simulink model "DLCReferenceApplication"  (R2018a)
settings: Solver=ode23tb  StartTime=0.0  StopTime=20  FixedStep=.001  RelTol=5e-3  EnableMultiTasking=on
StartFcn:
  | %tic
StopFcn:
  | %toc
model workspace (MAT data in the model file):
  A_mu = 10
  B_reff = 8.386
  Cz = 7766.25
  DCT_Param : struct (value not decoded)
  D_reff = 0.25826
  Downshift_Speeds = [9.5625 12.9375 16.3125 19.6875 23.0625 26.4375 29.8125 33.1875 36.5625 39.9375 43.3125 46.6875 ... (28 elements, 4x7)]
  Pedal_Positions = [0.1 0.4 0.5 0.9]
  SUS : struct (value not decoded)
  Upshift_Speeds = [12.9375 16.3125 19.6875 33 26.4375 29.8125 33.1875 52.5 39.9375 43.3125 46.6875 77.25 ... (28 elements, 4x7)]
  VEH : struct (value not decoded)
  V_o = 16.7
  V_xlow = 1
  WH : struct (value not decoded)
  a = 1.4
  alpha_max = 1.5
  alpha_min = -1.5
  b = 1.8
  c_zo = 209651
  epsilon = 0.1
  h = 0.134
  path : struct (value not decoded)
  pio = 220000
  q_Fcx = 0
  q_Fz2 = 15.4
  q_Fzy = 0
  q_reo = 0.9974
  q_sx1 = -0.007764
  q_sx10 = 0.2824
  q_sx11 = 5.349
  q_sx12 = 0
  q_sx13 = 0
  q_sx14 = 0
  q_sx2 = 1.1915
  q_sx3 = 0.013948
  q_sx4 = 4.912
  q_sx5 = 1.02
  q_sx6 = 22.83
  q_sx7 = 0.7104
  q_sx8 = -0.023393
  q_sx9 = 0.6581
  q_sy1 = 0.00702
  q_sy2 = 0
  q_sy3 = 0.001515
  q_sy4 = 8.514e-05
  q_sy5 = 0
  q_sy6 = 0
  q_sy7 = 0.9008
  q_sy8 = -0.4089
  q_v1 = 0.0007742
  q_v2 = 0.04667
  r_Bx1 = 12.531
  r_Bx2 = 9.532
  r_Bx3 = 0
  r_By1 = 10.615
  r_By2 = 7.705
  r_By3 = 3.433e-06
  r_By4 = 0
  r_Cx1 = 1.019
  r_Cy1 = 1.0585
  r_Ex1 = -0.4487
  r_Ex2 = -0.4726
  r_Ey1 = 0.3132
  r_Ey2 = 7.63e-06
  r_Hx1 = 0.0002374
  r_Hy1 = 0.011646
  r_Hy2 = 7.63e-06
  r_Vy1 = 0.05654
  r_Vy2 = 7.63e-06
  r_Vy3 = 0
  r_Vy4 = 99.9
  r_Vy5 = 2
  r_Vy6 = 15.814
  r_o = 0.3135
  vehWidth = 2
  w = 1
symbols that are objects in the model workspace (value not decoded): VEH
libraries: neural x286, simulink x5, sim3dlib x2, autolibutils x1, vehdynlibscenariocommon x1, vehdynlibdriver x1, vehdynlibviscommon x1
(part 3 of 13)

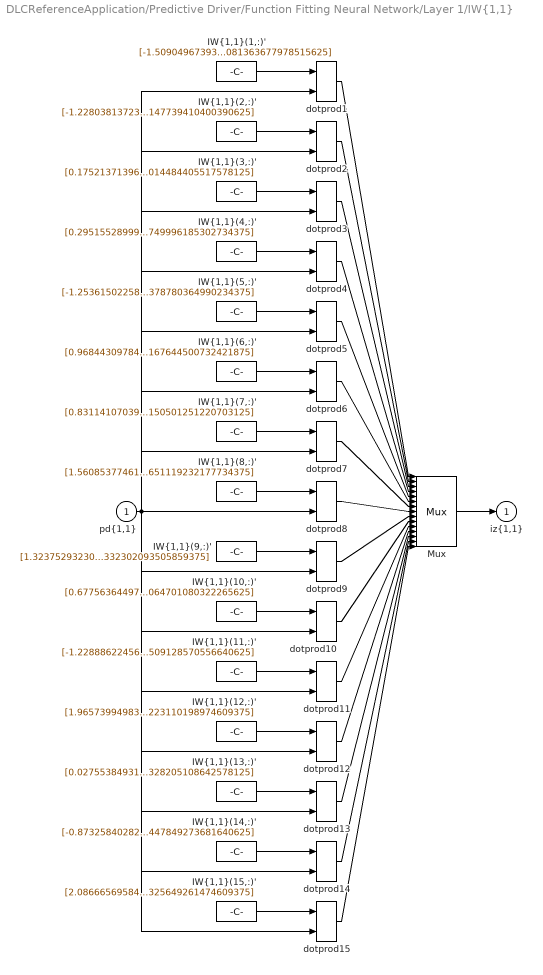
== system DLCReferenceApplication/Predictive Driver/Function Fitting Neural Network/Layer 1/IW{1,1} ==
  "pd{1,1}" : Inport  PortDimensions=7
      mask Display: e = 0.06;c1 = [120 230 180]/255;c2 = ([120 230 180]+0)/(256+128);c3 = ([120 230 180]+128)/(256+128);patch([0 1 1 0],[0 0 1 1],c1);patch([0 1 1 1-e 1-e 0+e],[0 0 1 1-e 0+e 0+e],c2);patch([0 0 1 1-e 0+e 0+e],[0 1 1 1-e 1-e 0+e],c3);plot([0 1 1 0 0],[0 0 1 1 0]);
  "IW{1,1}(1,:)'" : Constant  Value=[-1.509049673932340684956443510600365698337554931640625;1.51927734183694784775298103340901434421539306640625;1.479181269120346531309451165725477039813995361328125;0.76292036319028133650732570458785630762577056884765625;-1.4000753923386464183664656957262195646762847900390625;1.516189767355066830845089498325251042842864990234375;-0.6979172108090470061370069743134081363677978515625]
      mask Display: e = 0.06;c1 = [120 150 230]/255;c2 = ([120 150 230]+0)/383;c3 = ([120 150 230]+128)/383;patch([0 1 1 0],[0 0 1 1],c1);patch([0 1 1 1-e 1-e 0+e],[0 0 1 1-e 0+e 0+e],c2);patch([0 0 1 1-e 0+e 0+e],[0 1 1 1-e 1-e 0+e],c3);plot([0 1 1 0 0],[0 0 1 1 0]);disp('Weights');
  "IW{1,1}(10,:)'" : Constant  Value=[0.67756364497310739292146308798692189157009124755859375;0.04182033064572175662387820693766116164624691009521484375;-0.4504897562480543182772407817537896335124969482421875;-2.551876443899323110287014060304500162601470947265625;0.18672185850221978409280154664884321391582489013671875;1.7325835923135628480196146483649499714374542236328125;0.289998821125625971806272218600497581064701080322265625]
      mask Display: e = 0.06;c1 = [120 150 230]/255;c2 = ([120 150 230]+0)/383;c3 = ([120 150 230]+128)/383;patch([0 1 1 0],[0 0 1 1],c1);patch([0 1 1 1-e 1-e 0+e],[0 0 1 1-e 0+e 0+e],c2);patch([0 0 1 1-e 0+e 0+e],[0 1 1 1-e 1-e 0+e],c3);plot([0 1 1 0 0],[0 0 1 1 0]);disp('Weights');
  "IW{1,1}(11,:)'" : Constant  Value=[-1.2288862245678371376556015093228779733180999755859375;-0.70363000734339908870396129714208655059337615966796875;-1.5288499399296260339298214603331871330738067626953125;-1.1174320519343565738523693653405643999576568603515625;1.6750447749892007909267022114363498985767364501953125;-2.4972953199852252481605319189839065074920654296875;0.70182493954114166800906104981550015509128570556640625]
      mask Display: e = 0.06;c1 = [120 150 230]/255;c2 = ([120 150 230]+0)/383;c3 = ([120 150 230]+128)/383;patch([0 1 1 0],[0 0 1 1],c1);patch([0 1 1 1-e 1-e 0+e],[0 0 1 1-e 0+e 0+e],c2);patch([0 0 1 1-e 0+e 0+e],[0 1 1 1-e 1-e 0+e],c3);plot([0 1 1 0 0],[0 0 1 1 0]);disp('Weights');
  "IW{1,1}(12,:)'" : Constant  Value=[1.9657399498320062836143051754334010183811187744140625;0.055469671143939518198617832922536763362586498260498046875;0.428893001178795640893071094978949986398220062255859375;0.83038703202997699026610689543304033577442169189453125;0.6528646345537374440226585647906176745891571044921875;-1.7892558675957606073581018790719099342823028564453125;-1.87816849195586765830512376851402223110198974609375]
      mask Display: e = 0.06;c1 = [120 150 230]/255;c2 = ([120 150 230]+0)/383;c3 = ([120 150 230]+128)/383;patch([0 1 1 0],[0 0 1 1],c1);patch([0 1 1 1-e 1-e 0+e],[0 0 1 1-e 0+e 0+e],c2);patch([0 0 1 1-e 0+e 0+e],[0 1 1 1-e 1-e 0+e],c3);plot([0 1 1 0 0],[0 0 1 1 0]);disp('Weights');
  "IW{1,1}(13,:)'" : Constant  Value=[0.027553849311181564940564925336730084381997585296630859375;0.165556284993658930915216842549853026866912841796875;1.0787466889472050457499108233605511486530303955078125;-1.89957440383020159657689873711206018924713134765625;0.54115146920791890039481586427427828311920166015625;-1.653817387983281150809489190578460693359375;1.1876738967274527158934915860299952328205108642578125]
      mask Display: e = 0.06;c1 = [120 150 230]/255;c2 = ([120 150 230]+0)/383;c3 = ([120 150 230]+128)/383;patch([0 1 1 0],[0 0 1 1],c1);patch([0 1 1 1-e 1-e 0+e],[0 0 1 1-e 0+e 0+e],c2);patch([0 0 1 1-e 0+e 0+e],[0 1 1 1-e 1-e 0+e],c3);plot([0 1 1 0 0],[0 0 1 1 0]);disp('Weights');
  "IW{1,1}(14,:)'" : Constant  Value=[-0.873258402827774116161663187085650861263275146484375;2.211312160674173465935155036277137696743011474609375;-2.483318885241498463756215642206370830535888671875;2.537018816534186260724936801125295460224151611328125;2.2595527875997465372392980498261749744415283203125;-4.12440023174638614733567010262049734592437744140625;2.3447201728720248325998909422196447849273681640625]
      mask Display: e = 0.06;c1 = [120 150 230]/255;c2 = ([120 150 230]+0)/383;c3 = ([120 150 230]+128)/383;patch([0 1 1 0],[0 0 1 1],c1);patch([0 1 1 1-e 1-e 0+e],[0 0 1 1-e 0+e 0+e],c2);patch([0 0 1 1-e 0+e 0+e],[0 1 1 1-e 1-e 0+e],c3);plot([0 1 1 0 0],[0 0 1 1 0]);disp('Weights');
  "IW{1,1}(15,:)'" : Constant  Value=[2.08666569584865957409647307940758764743804931640625;-0.80442585468800620329687944831675849854946136474609375;-0.379133263113434482161068217465071938931941986083984375;-0.2375698497917715368288327226764522492885589599609375;0.10421540704451726089274643527460284531116485595703125;-0.77514844988269893111265673724119551479816436767578125;0.3039233762085336021385728599852882325649261474609375]
      mask Display: e = 0.06;c1 = [120 150 230]/255;c2 = ([120 150 230]+0)/383;c3 = ([120 150 230]+128)/383;patch([0 1 1 0],[0 0 1 1],c1);patch([0 1 1 1-e 1-e 0+e],[0 0 1 1-e 0+e 0+e],c2);patch([0 0 1 1-e 0+e 0+e],[0 1 1 1-e 1-e 0+e],c3);plot([0 1 1 0 0],[0 0 1 1 0]);disp('Weights');
  "IW{1,1}(2,:)'" : Constant  Value=[-1.22803813723280175196350683108903467655181884765625;-2.25896918882737285372286351048387587070465087890625;-0.4219079312453886121403456854750402271747589111328125;-1.695805476122420163420656535890884697437286376953125;1.6764860652005861840763145664823241531848907470703125;-0.288104929415635313549870488714077509939670562744140625;1.1836646212486352514048348893993534147739410400390625]
      mask Display: e = 0.06;c1 = [120 150 230]/255;c2 = ([120 150 230]+0)/383;c3 = ([120 150 230]+128)/383;patch([0 1 1 0],[0 0 1 1],c1);patch([0 1 1 1-e 1-e 0+e],[0 0 1 1-e 0+e 0+e],c2);patch([0 0 1 1-e 0+e 0+e],[0 1 1 1-e 1-e 0+e],c3);plot([0 1 1 0 0],[0 0 1 1 0]);disp('Weights');
  "IW{1,1}(3,:)'" : Constant  Value=[0.17521371396843898882167422925704158842563629150390625;-1.5068324243738988599261574563570320606231689453125;-0.339896798386482734688485152219072915613651275634765625;1.2475380308633063908274607456405647099018096923828125;3.277106824369047100020679863519035279750823974609375;0.1745122092133344626763147289238986559212207794189453125;-2.210738215368686088169170034234412014484405517578125]
      mask Display: e = 0.06;c1 = [120 150 230]/255;c2 = ([120 150 230]+0)/383;c3 = ([120 150 230]+128)/383;patch([0 1 1 0],[0 0 1 1],c1);patch([0 1 1 1-e 1-e 0+e],[0 0 1 1-e 0+e 0+e],c2);patch([0 0 1 1-e 0+e 0+e],[0 1 1 1-e 1-e 0+e],c3);plot([0 1 1 0 0],[0 0 1 1 0]);disp('Weights');
  "IW{1,1}(4,:)'" : Constant  Value=[0.295155289995136682623666501967818476259708404541015625;0.54169014463003517523276286738109774887561798095703125;-0.81923187750457915345947412788518704473972320556640625;-1.413502828991773707656420810963027179241180419921875;0.7249327311390978412219965321128256618976593017578125;0.25822608938690316815467440392239950597286224365234375;3.05246104088644099050497970893047749996185302734375]
      mask Display: e = 0.06;c1 = [120 150 230]/255;c2 = ([120 150 230]+0)/383;c3 = ([120 150 230]+128)/383;patch([0 1 1 0],[0 0 1 1],c1);patch([0 1 1 1-e 1-e 0+e],[0 0 1 1-e 0+e 0+e],c2);patch([0 0 1 1-e 0+e 0+e],[0 1 1 1-e 1-e 0+e],c3);plot([0 1 1 0 0],[0 0 1 1 0]);disp('Weights');
  "IW{1,1}(5,:)'" : Constant  Value=[-1.253615022589892991078386330627836287021636962890625;-1.308178888292455877007114395382814109325408935546875;-0.55746399823290404551556775913923047482967376708984375;2.888853599694045204415715488721616566181182861328125;0.67366408192522564402082707601948641240596771240234375;1.7511351672237738252846384057193063199520111083984375;-0.550561400887894958344759288593195378780364990234375]
      mask Display: e = 0.06;c1 = [120 150 230]/255;c2 = ([120 150 230]+0)/383;c3 = ([120 150 230]+128)/383;patch([0 1 1 0],[0 0 1 1],c1);patch([0 1 1 1-e 1-e 0+e],[0 0 1 1-e 0+e 0+e],c2);patch([0 0 1 1-e 0+e 0+e],[0 1 1 1-e 1-e 0+e],c3);plot([0 1 1 0 0],[0 0 1 1 0]);disp('Weights');
  "IW{1,1}(6,:)'" : Constant  Value=[0.968443097846008793538885583984665572643280029296875;-1.02085143200877492830613846308551728725433349609375;-2.7100181628849835391292799613438546657562255859375;-1.469426684764355339751773499301634728908538818359375;-0.72093283243393291304101921923574991524219512939453125;0.0298446565267905077056820317693563993088901042938232421875;0.2776436857395701007789057257468812167644500732421875]
      mask Display: e = 0.06;c1 = [120 150 230]/255;c2 = ([120 150 230]+0)/383;c3 = ([120 150 230]+128)/383;patch([0 1 1 0],[0 0 1 1],c1);patch([0 1 1 1-e 1-e 0+e],[0 0 1 1-e 0+e 0+e],c2);patch([0 0 1 1-e 0+e 0+e],[0 1 1 1-e 1-e 0+e],c3);plot([0 1 1 0 0],[0 0 1 1 0]);disp('Weights');
  "IW{1,1}(7,:)'" : Constant  Value=[0.83114107039691231815226046819589100778102874755859375;-1.653778663789594371991142907063476741313934326171875;1.7070538673297175336074360529892146587371826171875;-0.467894735272818274030015572861884720623493194580078125;-1.4874423762862181153110441300668753683567047119140625;0.1529353896317520999925676505881710909307003021240234375;-0.51792644395898801423783197606098838150501251220703125]
      mask Display: e = 0.06;c1 = [120 150 230]/255;c2 = ([120 150 230]+0)/383;c3 = ([120 150 230]+128)/383;patch([0 1 1 0],[0 0 1 1],c1);patch([0 1 1 1-e 1-e 0+e],[0 0 1 1-e 0+e 0+e],c2);patch([0 0 1 1-e 0+e 0+e],[0 1 1 1-e 1-e 0+e],c3);plot([0 1 1 0 0],[0 0 1 1 0]);disp('Weights');
  "IW{1,1}(8,:)'" : Constant  Value=[1.5608537746191044615073906243196688592433929443359375;0.8208342730039908108352619819925166666507720947265625;1.70216863375625049314976422465406358242034912109375;-0.95886390034983914887334321974776685237884521484375;3.42297237946134469410708334180526435375213623046875;0.6162829570883274765691339780460111796855926513671875;3.2692680483829601456591262831352651119232177734375]
      mask Display: e = 0.06;c1 = [120 150 230]/255;c2 = ([120 150 230]+0)/383;c3 = ([120 150 230]+128)/383;patch([0 1 1 0],[0 0 1 1],c1);patch([0 1 1 1-e 1-e 0+e],[0 0 1 1-e 0+e 0+e],c2);patch([0 0 1 1-e 0+e 0+e],[0 1 1 1-e 1-e 0+e],c3);plot([0 1 1 0 0],[0 0 1 1 0]);disp('Weights');
  "IW{1,1}(9,:)'" : Constant  Value=[1.3237529323020209570671568144462071359157562255859375;-0.44844324720964079400431501198909245431423187255859375;-3.795885956504914116038662541541270911693572998046875;-1.1322778939762268013424773016595281660556793212890625;-0.50600361676503669006166319377371110022068023681640625;-1.3597783903850106934640962208504788577556610107421875;-1.599955115091173496466581127606332302093505859375]
      mask Display: e = 0.06;c1 = [120 150 230]/255;c2 = ([120 150 230]+0)/383;c3 = ([120 150 230]+128)/383;patch([0 1 1 0],[0 0 1 1],c1);patch([0 1 1 1-e 1-e 0+e],[0 0 1 1-e 0+e 0+e],c2);patch([0 0 1 1-e 0+e 0+e],[0 1 1 1-e 1-e 0+e],c3);plot([0 1 1 0 0],[0 0 1 1 0]);disp('Weights');
  Mux : Mux  Inputs=15
      mask Display: e = 0.06;c1 = [120 150 230]/255;c2 = ([120 150 230]+0)/383;c3 = ([120 150 230]+128)/383;patch([0 1 1 0],[0 0 1 1],c1);patch([0 1 1 1-e 1-e 0+e],[0 0 1 1-e 0+e 0+e],c2);patch([0 0 1 1-e 0+e 0+e],[0 1 1 1-e 1-e 0+e],c3);plot([0 1 1 0 0],[0 0 1 1 0]);disp('Mux');
  dotprod{1..15} (15 alike) : neural/Weight Functions/dotprod
  "iz{1,1}" : Outport
      mask Display: e = 0.06;c1 = [120 230 180]/255;c2 = ([120 230 180]+0)/(256+128);c3 = ([120 230 180]+128)/(256+128);patch([0 1 1 0],[0 0 1 1],c1);patch([0 1 1 1-e 1-e 0+e],[0 0 1 1-e 0+e 0+e],c2);patch([0 0 1 1-e 0+e 0+e],[0 1 1 1-e 1-e 0+e],c3);plot([0 1 1 0 0],[0 0 1 1 0]);
  wires:
  "IW{1,1}(1,:)'"/1 -> dotprod1/1
  "pd{1,1}"/1 -> dotprod1/2, dotprod2/2, dotprod3/2, dotprod4/2, dotprod5/2, dotprod6/2, dotprod7/2, dotprod8/2, dotprod9/2, dotprod10/2, dotprod11/2, dotprod12/2, dotprod13/2, dotprod14/2, dotprod15/2
  dotprod1/1 -> Mux/1
  "IW{1,1}(2,:)'"/1 -> dotprod2/1
  dotprod2/1 -> Mux/2
  "IW{1,1}(3,:)'"/1 -> dotprod3/1
  dotprod3/1 -> Mux/3
  "IW{1,1}(4,:)'"/1 -> dotprod4/1
  dotprod4/1 -> Mux/4
  "IW{1,1}(5,:)'"/1 -> dotprod5/1
  dotprod5/1 -> Mux/5
  "IW{1,1}(6,:)'"/1 -> dotprod6/1
  dotprod6/1 -> Mux/6
  "IW{1,1}(7,:)'"/1 -> dotprod7/1
  dotprod7/1 -> Mux/7
  "IW{1,1}(8,:)'"/1 -> dotprod8/1
  dotprod8/1 -> Mux/8
  "IW{1,1}(9,:)'"/1 -> dotprod9/1
  dotprod9/1 -> Mux/9
  "IW{1,1}(10,:)'"/1 -> dotprod10/1
  dotprod10/1 -> Mux/10
  "IW{1,1}(11,:)'"/1 -> dotprod11/1
  dotprod11/1 -> Mux/11
  "IW{1,1}(12,:)'"/1 -> dotprod12/1
  dotprod12/1 -> Mux/12
  "IW{1,1}(13,:)'"/1 -> dotprod13/1
  dotprod13/1 -> Mux/13
  "IW{1,1}(14,:)'"/1 -> dotprod14/1
  dotprod14/1 -> Mux/14
  "IW{1,1}(15,:)'"/1 -> dotprod15/1
  dotprod15/1 -> Mux/15
  Mux/1 -> "iz{1,1}"/1

== system DLCReferenceApplication/Predictive Driver/Function Fitting Neural Network/Layer 2/Delays 1 ==
  "p{2}" : Inport  PortDimensions=15
      mask Display: e = 0.06;c1 = [120 230 180]/255;c2 = ([120 230 180]+0)/(256+128);c3 = ([120 230 180]+128)/(256+128);patch([0 1 1 0],[0 0 1 1],c1);patch([0 1 1 1-e 1-e 0+e],[0 0 1 1-e 0+e 0+e],c2);patch([0 0 1 1-e 0+e 0+e],[0 1 1 1-e 1-e 0+e],c3);plot([0 1 1 0 0],[0 0 1 1 0]);
  mux : Mux  Inputs=1
      mask Display: e = 0.06;c1 = [120 150 230]/255;c2 = ([120 150 230]+0)/383;c3 = ([120 150 230]+128)/383;patch([0 1 1 0],[0 0 1 1],c1);patch([0 1 1 1-e 1-e 0+e],[0 0 1 1-e 0+e 0+e],c2);patch([0 0 1 1-e 0+e 0+e],[0 1 1 1-e 1-e 0+e],c3);plot([0 1 1 0 0],[0 0 1 1 0]);disp('Mux')
  "pd{2,1}" : Outport
      mask Display: e = 0.06;c1 = [120 230 180]/255;c2 = ([120 230 180]+0)/(256+128);c3 = ([120 230 180]+128)/(256+128);patch([0 1 1 0],[0 0 1 1],c1);patch([0 1 1 1-e 1-e 0+e],[0 0 1 1-e 0+e 0+e],c2);patch([0 0 1 1-e 0+e 0+e],[0 1 1 1-e 1-e 0+e],c3);plot([0 1 1 0 0],[0 0 1 1 0]);
  wires:
  "p{2}"/1 -> mux/1
  mux/1 -> "pd{2,1}"/1

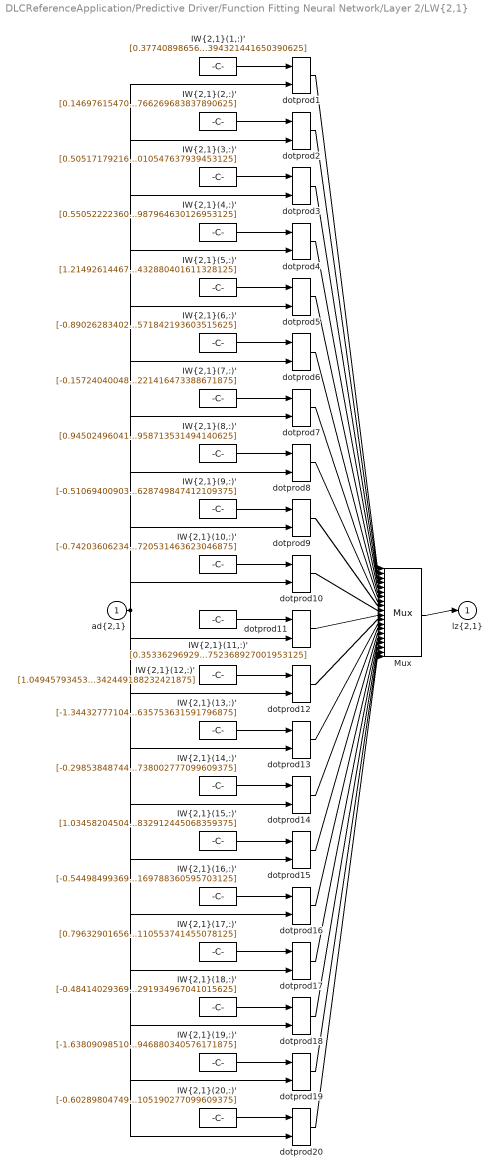
== system DLCReferenceApplication/Predictive Driver/Function Fitting Neural Network/Layer 2/LW{2,1} ==
  "ad{2,1}" : Inport  PortDimensions=15
      mask Display: e = 0.06;c1 = [120 230 180]/255;c2 = ([120 230 180]+0)/(256+128);c3 = ([120 230 180]+128)/(256+128);patch([0 1 1 0],[0 0 1 1],c1);patch([0 1 1 1-e 1-e 0+e],[0 0 1 1-e 0+e 0+e],c2);patch([0 0 1 1-e 0+e 0+e],[0 1 1 1-e 1-e 0+e],c3);plot([0 1 1 0 0],[0 0 1 1 0]);
  "IW{2,1}(1,:)'" : Constant  Value=[0.377408986567094262287724859561421908438205718994140625;0.916935828034818545262396582984365522861480712890625;0.393088948975864271861979659661301411688327789306640625;-0.6492111185444693344237521159811876714229583740234375;-0.203739226760496883184003991118515841662883758544921875;-0.1100086759278134651562908175037591718137264251708984375;0.351124696378162237664355416200123727321624755859375;0.540735910832136124071212179842405021190643310546875;-0.52499617358879613338018543799989856779575347900390625;-0.8542847095270953428070015434059314429759979248046875;0.7305202305645150939739096429548226296901702880859375;0.26047154767623614812777077531791292130947113037109375;-0.5187381603465672785802098587737418711185455322265625;0.11664270786766640919385196184521191753447055816650390625;-0.374314853750083609273957563345902599394321441650390625]
      mask Display: e = 0.06;c1 = [120 150 230]/255;c2 = ([120 150 230]+0)/383;c3 = ([120 150 230]+128)/383;patch([0 1 1 0],[0 0 1 1],c1);patch([0 1 1 1-e 1-e 0+e],[0 0 1 1-e 0+e 0+e],c2);patch([0 0 1 1-e 0+e 0+e],[0 1 1 1-e 1-e 0+e],c3);plot([0 1 1 0 0],[0 0 1 1 0]);disp('weights');
  "IW{2,1}(10,:)'" : Constant  Value=[-0.74203606234167496236153738209395669400691986083984375;-0.812696026932474335779943430679850280284881591796875;-0.6131789681735482222535438268096186220645904541015625;0.1180891377801421004978266182661172933876514434814453125;0.397427019878926424123477545435889624059200286865234375;2.659200302624636691462001181207597255706787109375;0.8379336594029853646503624986507929861545562744140625;-0.51262919422646213707395190795068629086017608642578125;-0.2688533984134124921183683909475803375244140625;0.7557158363858416105784954197588376700878143310546875;-0.492959648338735345607375393228721804916858673095703125;0.0773063422443649173043667133242706768214702606201171875;-0.406745691526066044385601117028272710740566253662109375;-0.7792669239456808671917542596929706633090972900390625;0.6259901693968170643955772902700118720531463623046875]
      mask Display: e = 0.06;c1 = [120 150 230]/255;c2 = ([120 150 230]+0)/383;c3 = ([120 150 230]+128)/383;patch([0 1 1 0],[0 0 1 1],c1);patch([0 1 1 1-e 1-e 0+e],[0 0 1 1-e 0+e 0+e],c2);patch([0 0 1 1-e 0+e 0+e],[0 1 1 1-e 1-e 0+e],c3);plot([0 1 1 0 0],[0 0 1 1 0]);disp('weights');
  "IW{2,1}(11,:)'" : Constant  Value=[0.3533629692989530557412081179791130125522613525390625;-0.81541740940325035946756315752281807363033294677734375;-2.0683095123156203243297568405978381633758544921875;0.35160466105935561653694776396150700747966766357421875;0.47449346143949344689616509640472941100597381591796875;1.85236410264457074248412027372978627681732177734375;-0.81173488668558591019319692350109107792377471923828125;-0.8655341239549638743255854933522641658782958984375;0.54966802080016818887742147126118652522563934326171875;0.0288250527353895273641182228629986639134585857391357421875;-0.51036540540294594858750087951193563640117645263671875;-0.040133000774815463795874848074163310229778289794921875;-0.89000331812890742799737608947907574474811553955078125;0.678463611178770964471596016664989292621612548828125;0.04549854251039338326467742490422097034752368927001953125]
      mask Display: e = 0.06;c1 = [120 150 230]/255;c2 = ([120 150 230]+0)/383;c3 = ([120 150 230]+128)/383;patch([0 1 1 0],[0 0 1 1],c1);patch([0 1 1 1-e 1-e 0+e],[0 0 1 1-e 0+e 0+e],c2);patch([0 0 1 1-e 0+e 0+e],[0 1 1 1-e 1-e 0+e],c3);plot([0 1 1 0 0],[0 0 1 1 0]);disp('weights');
  "IW{2,1}(12,:)'" : Constant  Value=[1.0494579345300130146512174178496934473514556884765625;1.3044889644552188912030032952316105365753173828125;-0.27106298353604463269306279471493326127529144287109375;-0.1915871026849610692099901143592433072626590728759765625;-0.34760653690221354761291649992926977574825286865234375;0.52037978849581134621615774449310265481472015380859375;-0.2321169942446153766635319470879039727151393890380859375;0.332861282582828821308140732071478851139545440673828125;-1.3938611465836869829360011863172985613346099853515625;0.8212779725642869177448801565333269536495208740234375;0.1046906705946868132439675491696107201278209686279296875;-0.30151606216337956123396679686265997588634490966796875;0.4956805530473360477117239497601985931396484375;-0.71076779296117820194922387599945068359375;-0.48071803830861703499266468497808091342449188232421875]
      mask Display: e = 0.06;c1 = [120 150 230]/255;c2 = ([120 150 230]+0)/383;c3 = ([120 150 230]+128)/383;patch([0 1 1 0],[0 0 1 1],c1);patch([0 1 1 1-e 1-e 0+e],[0 0 1 1-e 0+e 0+e],c2);patch([0 0 1 1-e 0+e 0+e],[0 1 1 1-e 1-e 0+e],c3);plot([0 1 1 0 0],[0 0 1 1 0]);disp('weights');
  "IW{2,1}(13,:)'" : Constant  Value=[-1.344327771042938213241768607986159622669219970703125;-0.349408651716258733532782798647531308233737945556640625;-0.390264497355393424893321707713766954839229583740234375;0.126088036555836335850244722678326070308685302734375;-2.274693199742918725547724534408189356327056884765625;0.91296441439649156368574267617077566683292388916015625;-0.68148198466500409242740943227545358240604400634765625;1.2270973965697422602971755623002536594867706298828125;1.630906495799371302979352549300529062747955322265625;0.264212234475461105187577004471677355468273162841796875;0.2189450303855997592705762144760228693485260009765625;0.174476426404878981468726806269842199981212615966796875;0.5415687999290670351371090873726643621921539306640625;2.03925215568979556479689563275314867496490478515625;0.609317467002977508627736824564635753631591796875]
      mask Display: e = 0.06;c1 = [120 150 230]/255;c2 = ([120 150 230]+0)/383;c3 = ([120 150 230]+128)/383;patch([0 1 1 0],[0 0 1 1],c1);patch([0 1 1 1-e 1-e 0+e],[0 0 1 1-e 0+e 0+e],c2);patch([0 0 1 1-e 0+e 0+e],[0 1 1 1-e 1-e 0+e],c3);plot([0 1 1 0 0],[0 0 1 1 0]);disp('weights');
  "IW{2,1}(14,:)'" : Constant  Value=[-0.29853848744158828498740376744535751640796661376953125;1.1233511551870878353298621732392348349094390869140625;-2.07527020696446840020144009031355381011962890625;-1.935997401690873420676552996155805885791778564453125;-1.6993223712170613115546302651637233793735504150390625;1.3212505337032693919496750822872854769229888916015625;0.7734893293394142776975286324159242212772369384765625;2.973096611283996271168916791793890297412872314453125;3.26010917906186392656309180893003940582275390625;-1.6677811408871558995770101319067180156707763671875;1.0701107857236877851647705028881318867206573486328125;-0.51453166722322707382630824213265441358089447021484375;0.08834850909999403256733785383403301239013671875;1.4147674075361222900681923420052044093608856201171875;-1.09341438015672220984697560197673738002777099609375]
      mask Display: e = 0.06;c1 = [120 150 230]/255;c2 = ([120 150 230]+0)/383;c3 = ([120 150 230]+128)/383;patch([0 1 1 0],[0 0 1 1],c1);patch([0 1 1 1-e 1-e 0+e],[0 0 1 1-e 0+e 0+e],c2);patch([0 0 1 1-e 0+e 0+e],[0 1 1 1-e 1-e 0+e],c3);plot([0 1 1 0 0],[0 0 1 1 0]);disp('weights');
  "IW{2,1}(15,:)'" : Constant  Value=[1.0345820450408365065442239938420243561267852783203125;0.170053385086431474437773658792139030992984771728515625;0.425304751501224875820383886093623004853725433349609375;1.7849387921699018111354462234885431826114654541015625;0.058793108846872381423320774729290860705077648162841796875;-0.687600743270277536822732145083136856555938720703125;1.0963569888999680213004239703877829015254974365234375;1.22901382704288497649258715682663023471832275390625;-0.51720567140802875538696525836712680757045745849609375;-1.3060344490884323587209792094654403626918792724609375;-0.1371645083842421286579593697751988656818866729736328125;1.1056048523673409622603003299445845186710357666015625;0.1806329461051024709572487836339860223233699798583984375;1.400960637981855771982964142807759344577789306640625;-0.107830010639707152275690305032185278832912445068359375]
      mask Display: e = 0.06;c1 = [120 150 230]/255;c2 = ([120 150 230]+0)/383;c3 = ([120 150 230]+128)/383;patch([0 1 1 0],[0 0 1 1],c1);patch([0 1 1 1-e 1-e 0+e],[0 0 1 1-e 0+e 0+e],c2);patch([0 0 1 1-e 0+e 0+e],[0 1 1 1-e 1-e 0+e],c3);plot([0 1 1 0 0],[0 0 1 1 0]);disp('weights');
  "IW{2,1}(16,:)'" : Constant  Value=[-0.54498499369304098660649060548166744410991668701171875;0.6799088542563989090439235951635055243968963623046875;-0.59241245747564919010841322233318351209163665771484375;0.384464409586843858246396621325402520596981048583984375;0.0893006313696689535408523852311191149055957794189453125;1.07254602817469635311908859875984489917755126953125;-0.11425203906562857170126079608962754718959331512451171875;0.338543401462091331222126200373168103396892547607421875;-1.20203035787867218431301807868294417858123779296875;1.1448318723634363092145349583006463944911956787109375;-0.62571823313789221021608000228297896683216094970703125;-0.81788370770947416144025510220672003924846649169921875;-0.61074522886524273967978615473839454352855682373046875;0.292266194936081580291187265174812637269496917724609375;0.1836613738434247633524165621565771289169788360595703125]
      mask Display: e = 0.06;c1 = [120 150 230]/255;c2 = ([120 150 230]+0)/383;c3 = ([120 150 230]+128)/383;patch([0 1 1 0],[0 0 1 1],c1);patch([0 1 1 1-e 1-e 0+e],[0 0 1 1-e 0+e 0+e],c2);patch([0 0 1 1-e 0+e 0+e],[0 1 1 1-e 1-e 0+e],c3);plot([0 1 1 0 0],[0 0 1 1 0]);disp('weights');
  "IW{2,1}(17,:)'" : Constant  Value=[0.79632901656177512705880872090347111225128173828125;-0.43876079818712165891980703236185945570468902587890625;0.5548335307676006689092673695995472371578216552734375;-0.55849152574337879162413855738122947514057159423828125;-0.461844332172288318805186690951813943684101104736328125;-0.427115163073199521903688946622423827648162841796875;1.311178922459931062149962599505670368671417236328125;-1.1444708041324578307040837898966856300830841064453125;-2.238224649663369092422726680524647235870361328125;-0.2468042015115130827229705801073578186333179473876953125;0.252820664750389390018625590528245083987712860107421875;-1.268889152813235998706886675790883600711822509765625;-0.460334475021429156971208840332110412418842315673828125;0.32404132820950071192100949701853096485137939453125;0.375878502055563779027380633124266751110553741455078125]
      mask Display: e = 0.06;c1 = [120 150 230]/255;c2 = ([120 150 230]+0)/383;c3 = ([120 150 230]+128)/383;patch([0 1 1 0],[0 0 1 1],c1);patch([0 1 1 1-e 1-e 0+e],[0 0 1 1-e 0+e 0+e],c2);patch([0 0 1 1-e 0+e 0+e],[0 1 1 1-e 1-e 0+e],c3);plot([0 1 1 0 0],[0 0 1 1 0]);disp('weights');
  "IW{2,1}(18,:)'" : Constant  Value=[-0.48414029369150057835469169731368310749530792236328125;0.2455425835334756612393647401404450647532939910888671875;2.175669169808506442365114708081819117069244384765625;-0.0169383857920981963085527155499221407808363437652587890625;1.7643193485798673858511165235540829598903656005859375;-0.1898086105258787181782054176437668502330780029296875;-0.33303470605840612694947822092217393219470977783203125;-3.475903204880608665661156919668428599834442138671875;-0.24847508074663904320544816073379479348659515380859375;-1.0674807523660112540397904012934304773807525634765625;-0.291036855408897843222604251423035748302936553955078125;0.6660233106397936975184848051867447793483734130859375;-1.421373196711812614267955723335035145282745361328125;-1.7621575028435054743880527894361875951290130615234375;-0.086594068381614930363099347232491709291934967041015625]
      mask Display: e = 0.06;c1 = [120 150 230]/255;c2 = ([120 150 230]+0)/383;c3 = ([120 150 230]+128)/383;patch([0 1 1 0],[0 0 1 1],c1);patch([0 1 1 1-e 1-e 0+e],[0 0 1 1-e 0+e 0+e],c2);patch([0 0 1 1-e 0+e 0+e],[0 1 1 1-e 1-e 0+e],c3);plot([0 1 1 0 0],[0 0 1 1 0]);disp('weights');
  "IW{2,1}(19,:)'" : Constant  Value=[-1.638090985101666507972595354658551514148712158203125;0.480827709429096028515004945802502334117889404296875;-1.4851154730728117758786765989498235285282135009765625;-0.9734283236699454722185009813983924686908721923828125;-0.21534839284540729931194391610915772616863250732421875;-0.94935571166668319964543343303375877439975738525390625;2.109650740065902585484991504927165806293487548828125;0.874642020436957157158985864953137934207916259765625;-0.4695084292603450837333411982399411499500274658203125;-0.00237264900648152810003210788636351935565471649169921875;0.356321045315291351496256311293109320104122161865234375;0.50368443540930629698237908087321557104587554931640625;-0.68205822623703882268131337696104310452938079833984375;-1.9020995948650292195480915324878878891468048095703125;0.70938452559907616556955645137350074946880340576171875]
      mask Display: e = 0.06;c1 = [120 150 230]/255;c2 = ([120 150 230]+0)/383;c3 = ([120 150 230]+128)/383;patch([0 1 1 0],[0 0 1 1],c1);patch([0 1 1 1-e 1-e 0+e],[0 0 1 1-e 0+e 0+e],c2);patch([0 0 1 1-e 0+e 0+e],[0 1 1 1-e 1-e 0+e],c3);plot([0 1 1 0 0],[0 0 1 1 0]);disp('weights');
  "IW{2,1}(2,:)'" : Constant  Value=[0.1469761547003029800162465789981069974601268768310546875;-0.578701316419981903749203411280177533626556396484375;0.341452645103678176230488361397874541580677032470703125;0.2386095773885203163988677488305256702005863189697265625;-0.36337242315637852119181161469896323978900909423828125;0.3665880503615490670910048720543272793292999267578125;-0.054700333175656763728955667147602071054279804229736328125;-0.57877376702347838044460104356403462588787078857421875;-0.551342495889702188804903926211409270763397216796875;0.23492513046047769353918965862249024212360382080078125;-0.239877000357964276222588750897557474672794342041015625;-0.5307654361972897749666344680008478462696075439453125;-0.5926226537027596830142783801420591771602630615234375;-0.37952698780855664839606333771371282637119293212890625;-0.77994410405117131634966654019081033766269683837890625]
      mask Display: e = 0.06;c1 = [120 150 230]/255;c2 = ([120 150 230]+0)/383;c3 = ([120 150 230]+128)/383;patch([0 1 1 0],[0 0 1 1],c1);patch([0 1 1 1-e 1-e 0+e],[0 0 1 1-e 0+e 0+e],c2);patch([0 0 1 1-e 0+e 0+e],[0 1 1 1-e 1-e 0+e],c3);plot([0 1 1 0 0],[0 0 1 1 0]);disp('weights');
  "IW{2,1}(20,:)'" : Constant  Value=[-0.60289804749850628429186372159165330231189727783203125;1.7330062937538868172993034022510983049869537353515625;1.573776484323565316714166328893043100833892822265625;0.2201108814813907688101579651629435829818248748779296875;-0.1919165645051046642510783613033709116280078887939453125;-1.547054173232626173017933979281224310398101806640625;-0.2912781093635989915213713175035081803798675537109375;2.68008493566688610343362597632221877574920654296875;1.8447874368568211167485060286708176136016845703125;-1.052293595326766695308151611243374645709991455078125;0.81899269464238944049583324158447794616222381591796875;0.76469669785111527016141508283908478915691375732421875;0.61962472738743501476932351579307578504085540771484375;1.41942268833172224873351296992041170597076416015625;-0.47486232672215356043210476855165325105190277099609375]
      mask Display: e = 0.06;c1 = [120 150 230]/255;c2 = ([120 150 230]+0)/383;c3 = ([120 150 230]+128)/383;patch([0 1 1 0],[0 0 1 1],c1);patch([0 1 1 1-e 1-e 0+e],[0 0 1 1-e 0+e 0+e],c2);patch([0 0 1 1-e 0+e 0+e],[0 1 1 1-e 1-e 0+e],c3);plot([0 1 1 0 0],[0 0 1 1 0]);disp('weights');
  "IW{2,1}(3,:)'" : Constant  Value=[0.50517179216705832001110820783651433885097503662109375;-0.59919078994797303483466066609253175556659698486328125;1.17889739811014404580191694549284875392913818359375;-0.004188677321987861745800074686485459096729755401611328125;1.0604996761056650900201248077792115509510040283203125;2.29707854769621544477331553935073316097259521484375;-1.0923530737408351232176073608570732176303863525390625;-1.3291304263570236088298770482651889324188232421875;-0.9265907227572416360317220096476376056671142578125;0.5675851564234577484313604145427234470844268798828125;-0.51406261460909485894177350928657688200473785400390625;0.900172666384182473819919323432259261608123779296875;0.99948624458061396946817467323853634297847747802734375;0.430866797028912451583693155043874867260456085205078125;0.4158939432728250285009607978281565010547637939453125]
      mask Display: e = 0.06;c1 = [120 150 230]/255;c2 = ([120 150 230]+0)/383;c3 = ([120 150 230]+128)/383;patch([0 1 1 0],[0 0 1 1],c1);patch([0 1 1 1-e 1-e 0+e],[0 0 1 1-e 0+e 0+e],c2);patch([0 0 1 1-e 0+e 0+e],[0 1 1 1-e 1-e 0+e],c3);plot([0 1 1 0 0],[0 0 1 1 0]);disp('weights');
  "IW{2,1}(4,:)'" : Constant  Value=[0.5505222236012532466276070408639498054981231689453125;1.951703456007682913053713491535745561122894287109375;-0.9897527108084924751807420761906541883945465087890625;0.89755279697985679288052551783039234578609466552734375;-0.324574947928065460356350513393408618867397308349609375;0.5752534850846224845355436627869494259357452392578125;1.3135611127646946716396314513985998928546905517578125;-0.9502825046618890159066950218402780592441558837890625;0.6522574358700186092363537682103924453258514404296875;0.5949410481339902911912531635607592761516571044921875;1.398497712690600192075862651108764111995697021484375;-0.013206755464696941226865334328977041877806186676025390625;0.46796638405616775013839969687978737056255340576171875;0.26359814804868531012971288873814046382904052734375;-0.1195916009349183017906881332237389869987964630126953125]
      mask Display: e = 0.06;c1 = [120 150 230]/255;c2 = ([120 150 230]+0)/383;c3 = ([120 150 230]+128)/383;patch([0 1 1 0],[0 0 1 1],c1);patch([0 1 1 1-e 1-e 0+e],[0 0 1 1-e 0+e 0+e],c2);patch([0 0 1 1-e 0+e 0+e],[0 1 1 1-e 1-e 0+e],c3);plot([0 1 1 0 0],[0 0 1 1 0]);disp('weights');
  "IW{2,1}(5,:)'" : Constant  Value=[1.214926144670938956693362342775799334049224853515625;-0.589383392185145904562659779912792146205902099609375;1.222907349879617466825720839551649987697601318359375;-0.165693908486424401615977330948226153850555419921875;2.380733171177626505965463366010226309299468994140625;1.0699740607363887878733521574758924543857574462890625;-0.8153826367841781053158456415985710918903350830078125;-1.946087785836152050933378632180392742156982421875;0.039950547868003651041934887189199798740446567535400390625;0.055206800536407620028089837660445482470095157623291015625;0.5249489304239336462387655046768486499786376953125;0.360193257277666045723663046373985707759857177734375;2.023059243255165284836039063520729541778564453125;-1.8958752496376884977280496968887746334075927734375;-0.0896437504560290421284918238598038442432880401611328125]
      mask Display: e = 0.06;c1 = [120 150 230]/255;c2 = ([120 150 230]+0)/383;c3 = ([120 150 230]+128)/383;patch([0 1 1 0],[0 0 1 1],c1);patch([0 1 1 1-e 1-e 0+e],[0 0 1 1-e 0+e 0+e],c2);patch([0 0 1 1-e 0+e 0+e],[0 1 1 1-e 1-e 0+e],c3);plot([0 1 1 0 0],[0 0 1 1 0]);disp('weights');
  "IW{2,1}(6,:)'" : Constant  Value=[-0.89026283402007511114106819150038063526153564453125;-2.1276489961269913209207516047172248363494873046875;-0.718725775341054085032510556629858911037445068359375;-1.4049413007122077967636641915305517613887786865234375;2.126218402185191980180434256908483803272247314453125;0.52509099498448141840611924635595642030239105224609375;-0.2171988856466122996824452684450079686939716339111328125;0.1142472625616868520115332330533419735729694366455078125;-0.316690923671161306263144297190592624247074127197265625;0.87226111168505993109789642403484322130680084228515625;0.8645834666137088841963986851624213159084320068359375;0.0031807574741656535581568743253910724888555705547332763671875;-1.609828508172801431186371701187454164028167724609375;-1.005035215231575573824329694616608321666717529296875;0.6284007014447026140402385863126255571842193603515625]
      mask Display: e = 0.06;c1 = [120 150 230]/255;c2 = ([120 150 230]+0)/383;c3 = ([120 150 230]+128)/383;patch([0 1 1 0],[0 0 1 1],c1);patch([0 1 1 1-e 1-e 0+e],[0 0 1 1-e 0+e 0+e],c2);patch([0 0 1 1-e 0+e 0+e],[0 1 1 1-e 1-e 0+e],c3);plot([0 1 1 0 0],[0 0 1 1 0]);disp('weights');
  "IW{2,1}(7,:)'" : Constant  Value=[-0.15724040048056597829173597347107715904712677001953125;-1.05278750497809081565492306253872811794281005859375;0.9040750931625753938902789741405285894870758056640625;0.94070892345154033531429149661562405526638031005859375;-0.46009379460067967304581770804361440241336822509765625;-1.23031803174596721106581753701902925968170166015625;-0.8300200073230570296800578944385051727294921875;0.302220939663446819256620301530347205698490142822265625;0.500491149907080767889056005515158176422119140625;1.251261208996579110674929324886761605739593505859375;-0.09437800263282768165051805908660753630101680755615234375;-0.662283587664204365097475601942278444766998291015625;0.45797730429839400567715301804128102958202362060546875;-0.385832799381119972981224464092520065605640411376953125;0.3047115752056708259942752192728221416473388671875]
      mask Display: e = 0.06;c1 = [120 150 230]/255;c2 = ([120 150 230]+0)/383;c3 = ([120 150 230]+128)/383;patch([0 1 1 0],[0 0 1 1],c1);patch([0 1 1 1-e 1-e 0+e],[0 0 1 1-e 0+e 0+e],c2);patch([0 0 1 1-e 0+e 0+e],[0 1 1 1-e 1-e 0+e],c3);plot([0 1 1 0 0],[0 0 1 1 0]);disp('weights');
  "IW{2,1}(8,:)'" : Constant  Value=[0.945024960415079107178826234303414821624755859375;-0.294075471019162149044490206506452523171901702880859375;-0.7029985120569912648846866431995294988155364990234375;-0.062855179229177438049447346202214248478412628173828125;-0.446927348752318265301397559596807695925235748291015625;-0.2162056312035481042688189745604177005589008331298828125;-0.861414220128228880213328011450357735157012939453125;0.249922441248228321963864573262981139123439788818359375;-2.151403544335645623419850380741991102695465087890625;-1.21736486318454151245305183692835271358489990234375;0.58213987769719410803048731395392678678035736083984375;-2.222490038809282086873508887947537004947662353515625;-0.234943984865448818322164470373536460101604461669921875;0.041707572739841790310233449190491228364408016204833984375;-1.5976912306991339907114024754264391958713531494140625]
      mask Display: e = 0.06;c1 = [120 150 230]/255;c2 = ([120 150 230]+0)/383;c3 = ([120 150 230]+128)/383;patch([0 1 1 0],[0 0 1 1],c1);patch([0 1 1 1-e 1-e 0+e],[0 0 1 1-e 0+e 0+e],c2);patch([0 0 1 1-e 0+e 0+e],[0 1 1 1-e 1-e 0+e],c3);plot([0 1 1 0 0],[0 0 1 1 0]);disp('weights');
  "IW{2,1}(9,:)'" : Constant  Value=[-0.5106940090357865447145968573749996721744537353515625;1.0882240534587903635355132792028598487377166748046875;-0.5668936775342794387455569449230097234249114990234375;-0.6211555230864871379736769085866399109363555908203125;-0.1736481411168747379658583440686925314366817474365234375;0.57637365312470334455241527393809519708156585693359375;-0.36364059015678418251837911157053895294666290283203125;2.069141925217436561723616250674240291118621826171875;1.0578916873998929215616726651205681264400482177734375;2.433371189191607442126041860319674015045166015625;2.113497521068234075158898122026585042476654052734375;-0.801697605944433622227052183006890118122100830078125;-0.2188729172702668090977340398239903151988983154296875;0.50582241373919234472822381576406769454479217529296875;-0.76139232426326619584955324171460233628749847412109375]
      mask Display: e = 0.06;c1 = [120 150 230]/255;c2 = ([120 150 230]+0)/383;c3 = ([120 150 230]+128)/383;patch([0 1 1 0],[0 0 1 1],c1);patch([0 1 1 1-e 1-e 0+e],[0 0 1 1-e 0+e 0+e],c2);patch([0 0 1 1-e 0+e 0+e],[0 1 1 1-e 1-e 0+e],c3);plot([0 1 1 0 0],[0 0 1 1 0]);disp('weights');
  Mux : Mux  Inputs=20
      mask Display: e = 0.06;c1 = [120 150 230]/255;c2 = ([120 150 230]+0)/383;c3 = ([120 150 230]+128)/383;patch([0 1 1 0],[0 0 1 1],c1);patch([0 1 1 1-e 1-e 0+e],[0 0 1 1-e 0+e 0+e],c2);patch([0 0 1 1-e 0+e 0+e],[0 1 1 1-e 1-e 0+e],c3);plot([0 1 1 0 0],[0 0 1 1 0]);disp('Mux');
  dotprod{1..20} (20 alike) : neural/Weight Functions/dotprod
  "lz{2,1}" : Outport
      mask Display: e = 0.06;c1 = [120 230 180]/255;c2 = ([120 230 180]+0)/(256+128);c3 = ([120 230 180]+128)/(256+128);patch([0 1 1 0],[0 0 1 1],c1);patch([0 1 1 1-e 1-e 0+e],[0 0 1 1-e 0+e 0+e],c2);patch([0 0 1 1-e 0+e 0+e],[0 1 1 1-e 1-e 0+e],c3);plot([0 1 1 0 0],[0 0 1 1 0]);
  wires:
  "IW{2,1}(1,:)'"/1 -> dotprod1/1
  "ad{2,1}"/1 -> dotprod1/2, dotprod2/2, dotprod3/2, dotprod4/2, dotprod5/2, dotprod6/2, dotprod7/2, dotprod8/2, dotprod9/2, dotprod10/2, dotprod11/2, dotprod12/2, dotprod13/2, dotprod14/2, dotprod15/2, dotprod16/2, dotprod17/2, dotprod18/2, dotprod19/2, dotprod20/2
  dotprod1/1 -> Mux/1
  "IW{2,1}(2,:)'"/1 -> dotprod2/1
  dotprod2/1 -> Mux/2
  "IW{2,1}(3,:)'"/1 -> dotprod3/1
  dotprod3/1 -> Mux/3
  "IW{2,1}(4,:)'"/1 -> dotprod4/1
  dotprod4/1 -> Mux/4
  "IW{2,1}(5,:)'"/1 -> dotprod5/1
  dotprod5/1 -> Mux/5
  "IW{2,1}(6,:)'"/1 -> dotprod6/1
  dotprod6/1 -> Mux/6
  "IW{2,1}(7,:)'"/1 -> dotprod7/1
  dotprod7/1 -> Mux/7
  "IW{2,1}(8,:)'"/1 -> dotprod8/1
  dotprod8/1 -> Mux/8
  "IW{2,1}(9,:)'"/1 -> dotprod9/1
  dotprod9/1 -> Mux/9
  "IW{2,1}(10,:)'"/1 -> dotprod10/1
  dotprod10/1 -> Mux/10
  "IW{2,1}(11,:)'"/1 -> dotprod11/1
  dotprod11/1 -> Mux/11
  "IW{2,1}(12,:)'"/1 -> dotprod12/1
  dotprod12/1 -> Mux/12
  "IW{2,1}(13,:)'"/1 -> dotprod13/1
  dotprod13/1 -> Mux/13
  "IW{2,1}(14,:)'"/1 -> dotprod14/1
  dotprod14/1 -> Mux/14
  "IW{2,1}(15,:)'"/1 -> dotprod15/1
  dotprod15/1 -> Mux/15
  "IW{2,1}(16,:)'"/1 -> dotprod16/1
  dotprod16/1 -> Mux/16
  "IW{2,1}(17,:)'"/1 -> dotprod17/1
  dotprod17/1 -> Mux/17
  "IW{2,1}(18,:)'"/1 -> dotprod18/1
  dotprod18/1 -> Mux/18
  "IW{2,1}(19,:)'"/1 -> dotprod19/1
  dotprod19/1 -> Mux/19
  "IW{2,1}(20,:)'"/1 -> dotprod20/1
  dotprod20/1 -> Mux/20
  Mux/1 -> "lz{2,1}"/1

== system DLCReferenceApplication/Predictive Driver/Function Fitting Neural Network/Layer 3/Delays 1 ==
  "p{3}" : Inport  PortDimensions=20
      mask Display: e = 0.06;c1 = [120 230 180]/255;c2 = ([120 230 180]+0)/(256+128);c3 = ([120 230 180]+128)/(256+128);patch([0 1 1 0],[0 0 1 1],c1);patch([0 1 1 1-e 1-e 0+e],[0 0 1 1-e 0+e 0+e],c2);patch([0 0 1 1-e 0+e 0+e],[0 1 1 1-e 1-e 0+e],c3);plot([0 1 1 0 0],[0 0 1 1 0]);
  mux : Mux  Inputs=1
      mask Display: e = 0.06;c1 = [120 150 230]/255;c2 = ([120 150 230]+0)/383;c3 = ([120 150 230]+128)/383;patch([0 1 1 0],[0 0 1 1],c1);patch([0 1 1 1-e 1-e 0+e],[0 0 1 1-e 0+e 0+e],c2);patch([0 0 1 1-e 0+e 0+e],[0 1 1 1-e 1-e 0+e],c3);plot([0 1 1 0 0],[0 0 1 1 0]);disp('Mux')
  "pd{3,2}" : Outport
      mask Display: e = 0.06;c1 = [120 230 180]/255;c2 = ([120 230 180]+0)/(256+128);c3 = ([120 230 180]+128)/(256+128);patch([0 1 1 0],[0 0 1 1],c1);patch([0 1 1 1-e 1-e 0+e],[0 0 1 1-e 0+e 0+e],c2);patch([0 0 1 1-e 0+e 0+e],[0 1 1 1-e 1-e 0+e],c3);plot([0 1 1 0 0],[0 0 1 1 0]);
  wires:
  "p{3}"/1 -> mux/1
  mux/1 -> "pd{3,2}"/1
